simulink model "Block_PDFF_XZ_Ccode"  (R2017b)
settings: Solver=VariableStepAuto  StartTime=0.0  StopTime=Reference_time  RelTol=1e-3
values from neighbouring files (symbols this model uses):
  F_x = 5.975    [main_pdff.m]
  F_z = 4.955    [main_pdff.m]
  Kd_x = 4    [main_pdff.m]
  Kd_z = 4    [main_pdff.m]
  Kp_x = 460    [main_pdff.m]
  Kp_z = 355    [main_pdff.m]
undefined symbols (not defined in the file or in its folder): plantX, plantZ, Ts, Vmax
libraries: slctrlblks x1
settings Model: Creator=LAB816  LastModifiedBy=LAB_JHU

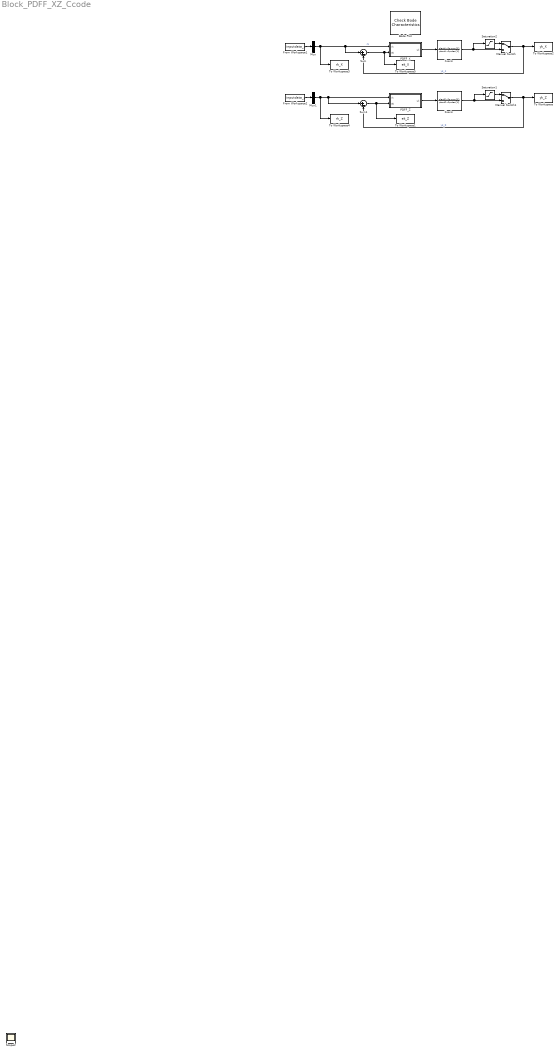
== system Block_PDFF_XZ_Ccode ==
  Bode Plot : slctrlblks/Model Verification/Check Bode  Characteristics  InstantiateOnLoad=on  SaveOperatingPoints=off  LinearizationIOs={'/Mux', 1, 'in', 'on', '';'/Manual Switch', 1, 'out', 'on', ''}  LinearizeAt=SnapshotTimes  SnapshotTimes=[0]  TriggerType=rising  SampleTime=auto  RateConversionMethod=zoh  PreWarpFreq=10  UseExactDelayModel=off  UseFullBlockNameLabels=off  UseBusSignalLabels=off  enabled=on  stopWhenAssertionFail=off  export=off  ViewDlgPos=[464 175 938 557]  OpenViewOnLoad=off  LaunchViewOnOpen=off  FrequencyUnits=rad/s  MagnitudeUnits=dB  PhaseUnits=deg  TimeUnits=seconds  EnableUpperBound=off  UpperBoundFrequencies=[]  UpperBoundMagnitudes=[]  EnableLowerBound=off  LowerBoundFrequencies=[]  LowerBoundMagnitudes=[]
      settings: SourceProductName=Simulink Control Design
  From Workspace1 : FromWorkspace  VariableName=inputdata_x  SampleTime=Ts
  From Workspace2 : FromWorkspace  VariableName=inputdata_z  SampleTime=Ts
  Manual Switch : ManualSwitch
  Manual Switch1 : ManualSwitch
  Mux : Mux  Inputs=1
  Mux1 : Mux  Inputs=1
  PDFF_X : Subsystem
  PDFF_Z : Subsystem
  Saturation1 : Saturate  UpperLimit=Vmax  LowerLimit=-Vmax
  Saturation2 : Saturate  UpperLimit=Vmax  LowerLimit=-Vmax
  Sum : Sum  Inputs=|+-
  Sum1 : Sum  Inputs=|+-
  To Workspace : ToWorkspace  VariableName=yk_Z  SampleTime=-1
  To Workspace1 : ToWorkspace  VariableName=ek_Z  SampleTime=-1
  To Workspace2 : ToWorkspace  VariableName=yk_X  SampleTime=-1
  To Workspace3 : ToWorkspace  VariableName=rk_X  SampleTime=-1
  To Workspace4 : ToWorkspace  VariableName=rk_Z  SampleTime=-1
  To Workspace5 : ToWorkspace  VariableName=ek_X  SampleTime=-1
  X-axis : DiscreteFilter  Numerator=plantX.v2p.num{1}  Denominator=plantX.v2p.den{1}  SampleTime=Ts
  Z-axis : DiscreteFilter  Numerator=plantZ.v2p.num{1}  Denominator=plantZ.v2p.den{1}  SampleTime=Ts
  Scope2 : Scope
  wires:
  PDFF_X/1(uk) -> X-axis/1
  Mux/1 -> To Workspace3/1, Sum/1, PDFF_X/1(rk)  "rk"
  Saturation2/1 -> Manual Switch/1
  X-axis/1 -> Manual Switch/2, Saturation2/1
  Manual Switch/1 -> Sum/2, To Workspace2/1  "yk_X"
  Saturation1/1 -> Manual Switch1/1
  Manual Switch1/1 -> To Workspace/1, Sum1/2  "yk_Z"
  Z-axis/1 -> Saturation1/1, Manual Switch1/2
  From Workspace1/1 -> Mux/1
  Sum1/1 -> To Workspace1/1, PDFF_Z/2(ek)
  PDFF_Z/1(uk) -> Z-axis/1
  Sum/1 -> To Workspace5/1, PDFF_X/2(ek)
  Mux1/1 -> To Workspace4/1, Sum1/1, PDFF_Z/1(rk)
  From Workspace2/1 -> Mux1/1

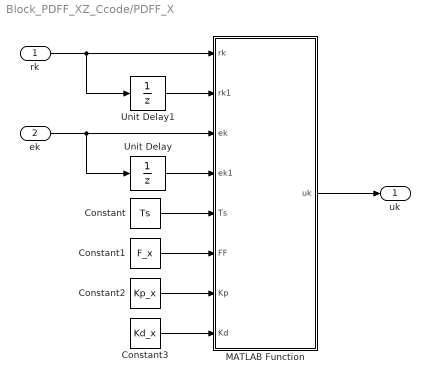
== system Block_PDFF_XZ_Ccode/PDFF_X ==
  rk : Inport
  ek : Inport  Port=2
  Constant : Constant  Value=Ts
  Constant1 : Constant  Value=F_x
  Constant2 : Constant  Value=Kp_x
  Constant3 : Constant  Value=Kd_x
  MATLAB Function : MATLAB Function  TreatAsAtomicUnit=on
  Unit Delay : UnitDelay  SampleTime=-1
  Unit Delay1 : UnitDelay  SampleTime=-1
  uk : Outport
  wires:
  Constant3/1 -> MATLAB Function/8(Kd)
  Constant2/1 -> MATLAB Function/7(Kp)
  Constant1/1 -> MATLAB Function/6(FF)
  ek/1 -> MATLAB Function/3(ek), Unit Delay/1
  rk/1 -> MATLAB Function/1(rk), Unit Delay1/1
  MATLAB Function/1(uk) -> uk/1
  Unit Delay/1 -> MATLAB Function/4(ek1)
  Unit Delay1/1 -> MATLAB Function/2(rk1)
  Constant/1 -> MATLAB Function/5(Ts)

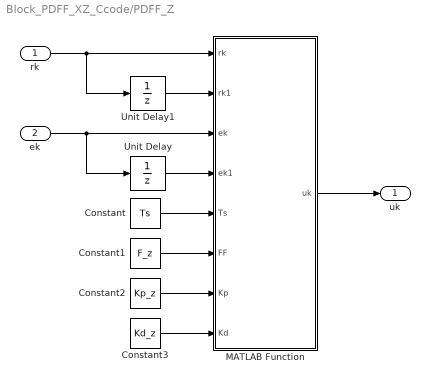
== system Block_PDFF_XZ_Ccode/PDFF_Z ==
  rk : Inport
  ek : Inport  Port=2
  Constant : Constant  Value=Ts
  Constant1 : Constant  Value=F_z
  Constant2 : Constant  Value=Kp_z
  Constant3 : Constant  Value=Kd_z
  MATLAB Function : MATLAB Function  TreatAsAtomicUnit=on
  Unit Delay : UnitDelay  SampleTime=-1
  Unit Delay1 : UnitDelay  SampleTime=-1
  uk : Outport
  wires:
  Constant/1 -> MATLAB Function/5(Ts)
  Unit Delay1/1 -> MATLAB Function/2(rk1)
  Unit Delay/1 -> MATLAB Function/4(ek1)
  MATLAB Function/1(uk) -> uk/1
  rk/1 -> Unit Delay1/1, MATLAB Function/1(rk)
  ek/1 -> Unit Delay/1, MATLAB Function/3(ek)
  Constant1/1 -> MATLAB Function/6(FF)
  Constant2/1 -> MATLAB Function/7(Kp)
  Constant3/1 -> MATLAB Function/8(Kd)

== matlab function Block_PDFF_XZ_Ccode/PDFF_X/MATLAB Function ==
  data: rk input; uk output; rk1 input; ek input; ek1 input; Ts input; FF input; Kp input; Kd input
function uk = PDFF_x(rk,rk1,ek,ek1,Ts,FF,Kp,Kd)    
    uk = FF*(rk-rk1)/Ts + Kp*ek + Kd*(ek-ek1)/Ts;
end

== matlab function Block_PDFF_XZ_Ccode/PDFF_Z/MATLAB Function ==
  data: rk input; uk output; rk1 input; ek input; ek1 input; Ts input; FF input; Kp input; Kd input
function uk = PDFF_z(rk,rk1,ek,ek1,Ts,FF,Kp,Kd)    
    uk = FF*(rk-rk1)/Ts + Kp*ek + Kd*(ek-ek1)/Ts;
end
